simulink model "simulacion"  (R2015a)
settings: Solver=ode45  StartTime=0.0  StopTime=3  RelTol=1e-3
settings Model: Creator=Jesus  LastModifiedBy=Jesus

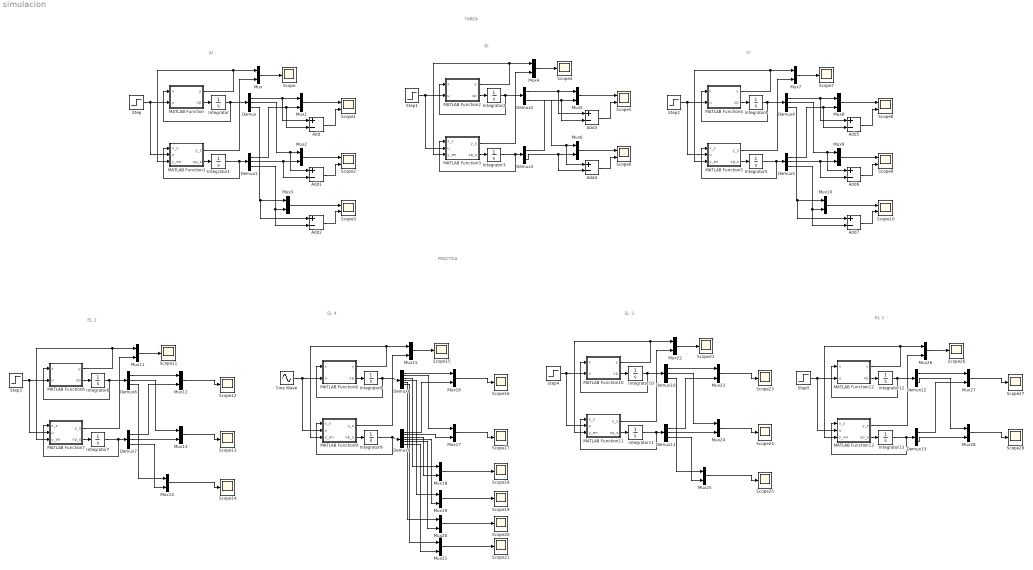
== system simulacion ==
  note: EJ. 4
  note: EJ. 2
  note: PRACTICA
  note: TAREA
  note: A)
  note: B)
  note: C)
  note: EJ. 3
  note: EJ. 1
  Add{,1..7} (8 alike) : Sum  Inputs=+-
  Demux{,1,4..7,10..11} (8 alike) : Demux  Outputs=3
  Demux{2..3,12..13} (4 alike) : Demux  Outputs=2
  Demux8 : Demux  Outputs=6
  Demux9 : Demux  Outputs=6
  Integrator : Integrator  InitialCondition=[3 2 5]
  Integrator{1,5,7,11} (4 alike) : Integrator  InitialCondition=[0 0 0]
  Integrator10 : Integrator  InitialCondition=[3 2 5]
  Integrator12 : Integrator  InitialCondition=[3 5]
  Integrator13 : Integrator  InitialCondition=[0 0]
  Integrator2 : Integrator  InitialCondition=[4 5]
  Integrator3 : Integrator  InitialCondition=[0 0]
  Integrator4 : Integrator  InitialCondition=[10 6 20]
  Integrator6 : Integrator  InitialCondition=[3 2 5]
  Integrator8 : Integrator  InitialCondition=[3 2 5 1 2 3]
  Integrator9 : Integrator  InitialCondition=[0 0 0 0 0 0]
  MATLAB Function : MATLAB Function  TreatAsAtomicUnit=on
  MATLAB Function1 : MATLAB Function  TreatAsAtomicUnit=on
  MATLAB Function10 : MATLAB Function  TreatAsAtomicUnit=on
  MATLAB Function11 : MATLAB Function  TreatAsAtomicUnit=on
  MATLAB Function12 : MATLAB Function  TreatAsAtomicUnit=on
  MATLAB Function13 : MATLAB Function  TreatAsAtomicUnit=on
  MATLAB Function2 : MATLAB Function  TreatAsAtomicUnit=on
  MATLAB Function3 : MATLAB Function  TreatAsAtomicUnit=on
  MATLAB Function4 : MATLAB Function  TreatAsAtomicUnit=on
  MATLAB Function5 : MATLAB Function  TreatAsAtomicUnit=on
  MATLAB Function6 : MATLAB Function  TreatAsAtomicUnit=on
  MATLAB Function7 : MATLAB Function  TreatAsAtomicUnit=on
  MATLAB Function8 : MATLAB Function  TreatAsAtomicUnit=on
  MATLAB Function9 : MATLAB Function  TreatAsAtomicUnit=on
  Mux{,1..28} (29 alike) : Mux  Inputs=2
  Scope{,4,7,11..28} (21 alike) : Scope
      Scope11 settings: SaveName=ScopeData11
      Scope12 settings: SaveName=ScopeData12
      Scope13 settings: SaveName=ScopeData13
      Scope14 settings: SaveName=ScopeData14
      Scope15 settings: SaveName=ScopeData15
      Scope16 settings: SaveName=ScopeData16
      Scope17 settings: YMin=-500000  YMax=5e+06  SaveName=ScopeData17
      Scope18 settings: YMin=-5000  YMax=5000  SaveName=ScopeData18
      Scope19 settings: YMin=-5000  YMax=5000  SaveName=ScopeData19
      Scope20 settings: YMin=-5000  YMax=5000  SaveName=ScopeData20
      Scope21 settings: YMin=-5000  YMax=5000  SaveName=ScopeData21
      Scope22 settings: SaveName=ScopeData22
      Scope23 settings: SaveName=ScopeData23
      Scope24 settings: SaveName=ScopeData24
      Scope25 settings: SaveName=ScopeData25
      Scope26 settings: SaveName=ScopeData26
      Scope27 settings: SaveName=ScopeData27
      Scope28 settings: SaveName=ScopeData28
      Scope4 settings: SaveName=ScopeData4
      Scope7 settings: SaveName=ScopeData8
  Scope{1..3,5..6,8..10} (8 alike) : Scope  NumInputPorts=2
      Scope1 settings: YMin=-5~-5  YMax=5~5
      Scope10 settings: YMin=-5~-5  YMax=5~5  SaveName=ScopeData7
      Scope2 settings: YMin=-5~-5  YMax=5~5  SaveName=ScopeData2
      Scope3 settings: YMin=-5~-5  YMax=5~5  SaveName=ScopeData3
      Scope5 settings: YMin=-5~-5  YMax=5~5  SaveName=ScopeData5
      Scope6 settings: YMin=-5~-5  YMax=5~5  SaveName=ScopeData6
      Scope8 settings: YMin=-5~-5  YMax=5~5  SaveName=ScopeData9
      Scope9 settings: YMin=-5~-5  YMax=5~5  SaveName=ScopeData10
  Sine Wave : Sin  Amplitude=5  SampleTime=0
  Step : Step  SampleTime=0
  Step1 : Step  SampleTime=0
  Step2 : Step  SampleTime=0
  Step3 : Step  After=10  SampleTime=0
  Step4 : Step  After=10  SampleTime=0
  Step5 : Step  After=10  SampleTime=0
  wires:
  MATLAB Function/2(xp) -> Integrator/1
  Integrator/1 -> Demux/1, MATLAB Function/1(x)
  Mux/1 -> Scope/1
  MATLAB Function/1(y) -> MATLAB Function1/3(y_en), Mux/1
  Step/1 -> MATLAB Function1/2(u), MATLAB Function/2(u)
  MATLAB Function1/2(xp_s) -> Integrator1/1
  Integrator1/1 -> MATLAB Function1/1(x_s), Demux1/1
  MATLAB Function1/1(y_s) -> Mux/2
  Demux/1 -> Add/1, Mux1/1
  Demux1/1 -> Add/2, Mux1/2
  Mux1/1 -> Scope1/1
  Mux2/1 -> Scope2/1
  Mux3/1 -> Scope3/1
  Demux/2 -> Add1/1, Mux2/1
  Demux1/2 -> Add1/2, Mux2/2
  Demux/3 -> Add2/1, Mux3/1
  Demux1/3 -> Add2/2, Mux3/2
  Add/1 -> Scope1/2
  Add2/1 -> Scope3/2
  Add1/1 -> Scope2/2
  MATLAB Function2/2(xp) -> Integrator2/1
  Integrator2/1 -> MATLAB Function2/1(x), Demux2/1
  Mux4/1 -> Scope4/1
  MATLAB Function2/1(y) -> Mux4/1, MATLAB Function3/3(y_en)
  Step1/1 -> MATLAB Function2/2(u), MATLAB Function3/2(u)
  MATLAB Function3/2(xp_s) -> Integrator3/1
  Integrator3/1 -> Demux3/1, MATLAB Function3/1(x_s)
  MATLAB Function3/1(y_s) -> Mux4/2
  Demux2/1 -> Mux5/1, Add3/1
  Demux3/1 -> Mux5/2, Add3/2
  Mux5/1 -> Scope5/1
  Mux6/1 -> Scope6/1
  Demux2/2 -> Mux6/1, Add4/1
  Demux3/2 -> Mux6/2, Add4/2
  Add3/1 -> Scope5/2
  Add4/1 -> Scope6/2
  MATLAB Function4/2(xp) -> Integrator4/1
  Integrator4/1 -> MATLAB Function4/1(x), Demux4/1
  Mux7/1 -> Scope7/1
  MATLAB Function4/1(y) -> Mux7/1, MATLAB Function5/3(y_en)
  Step2/1 -> MATLAB Function4/2(u), MATLAB Function5/2(u)
  MATLAB Function5/2(xp_s) -> Integrator5/1
  Integrator5/1 -> Demux5/1, MATLAB Function5/1(x_s)
  MATLAB Function5/1(y_s) -> Mux7/2
  Demux4/1 -> Mux8/1, Add5/1
  Demux5/1 -> Mux8/2, Add5/2
  Mux8/1 -> Scope8/1
  Mux9/1 -> Scope9/1
  Mux10/1 -> Scope10/1
  Demux4/2 -> Mux9/1, Add6/1
  Demux5/2 -> Mux9/2, Add6/2
  Demux4/3 -> Mux10/1, Add7/1
  Demux5/3 -> Mux10/2, Add7/2
  Add5/1 -> Scope8/2
  Add7/1 -> Scope10/2
  Add6/1 -> Scope9/2
  MATLAB Function6/2(xp) -> Integrator6/1
  Integrator6/1 -> MATLAB Function6/1(x), Demux6/1
  Mux11/1 -> Scope11/1
  MATLAB Function6/1(y) -> Mux11/1, MATLAB Function7/3(y_en)
  Step3/1 -> MATLAB Function6/2(u), MATLAB Function7/2(u)
  MATLAB Function7/2(xp_s) -> Integrator7/1
  Integrator7/1 -> Demux7/1, MATLAB Function7/1(x_s)
  MATLAB Function7/1(y_s) -> Mux11/2
  Demux6/1 -> Mux12/1
  Demux7/1 -> Mux12/2
  Mux12/1 -> Scope12/1
  Mux13/1 -> Scope13/1
  Mux14/1 -> Scope14/1
  Demux6/2 -> Mux13/1
  Demux7/2 -> Mux13/2
  Demux6/3 -> Mux14/1
  Demux7/3 -> Mux14/2
  MATLAB Function8/2(xp) -> Integrator8/1
  Integrator8/1 -> Demux8/1, MATLAB Function8/1(x)
  Mux15/1 -> Scope15/1
  MATLAB Function8/1(y) -> MATLAB Function9/3(y_en), Mux15/1
  Sine Wave/1 -> MATLAB Function9/2(u), MATLAB Function8/2(u)
  MATLAB Function9/2(xp_s) -> Integrator9/1
  Integrator9/1 -> MATLAB Function9/1(x_s), Demux9/1
  MATLAB Function9/1(y_s) -> Mux15/2
  Demux8/1 -> Mux16/1
  Demux9/1 -> Mux16/2
  Mux16/1 -> Scope16/1
  Mux17/1 -> Scope17/1
  Mux18/1 -> Scope18/1
  Demux8/2 -> Mux17/1
  Demux9/2 -> Mux17/2
  Demux8/3 -> Mux18/1
  Mux19/1 -> Scope19/1
  Demux8/4 -> Mux19/1
  Demux9/3 -> Mux18/2
  Demux9/4 -> Mux19/2
  Mux20/1 -> Scope20/1
  Demux8/5 -> Mux20/1
  Demux9/5 -> Mux20/2
  Mux21/1 -> Scope21/1
  Demux8/6 -> Mux21/1
  Demux9/6 -> Mux21/2
  MATLAB Function10/2(xp) -> Integrator10/1
  Integrator10/1 -> Demux10/1, MATLAB Function10/1(x)
  Mux22/1 -> Scope22/1
  MATLAB Function10/1(y) -> MATLAB Function11/3(y_en), Mux22/1
  Step4/1 -> MATLAB Function11/2(u), MATLAB Function10/2(u)
  MATLAB Function11/2(xp_s) -> Integrator11/1
  Integrator11/1 -> MATLAB Function11/1(x_s), Demux11/1
  MATLAB Function11/1(y_s) -> Mux22/2
  Demux10/1 -> Mux23/1
  Demux11/1 -> Mux23/2
  Mux23/1 -> Scope23/1
  Mux24/1 -> Scope24/1
  Mux25/1 -> Scope25/1
  Demux10/2 -> Mux24/1
  Demux11/2 -> Mux24/2
  Demux10/3 -> Mux25/1
  Demux11/3 -> Mux25/2
  MATLAB Function12/2(xp) -> Integrator12/1
  Integrator12/1 -> MATLAB Function12/1(x), Demux12/1
  Mux26/1 -> Scope26/1
  MATLAB Function12/1(y) -> Mux26/1, MATLAB Function13/3(y_en)
  Step5/1 -> MATLAB Function12/2(u), MATLAB Function13/2(u)
  MATLAB Function13/2(xp_s) -> Integrator13/1
  Integrator13/1 -> Demux13/1, MATLAB Function13/1(x_s)
  MATLAB Function13/1(y_s) -> Mux26/2
  Demux12/1 -> Mux27/1
  Demux13/1 -> Mux27/2
  Mux27/1 -> Scope27/1
  Mux28/1 -> Scope28/1
  Demux12/2 -> Mux28/1
  Demux13/2 -> Mux28/2

== matlab function simulacion/MATLAB Function1 ==
  data: x_s input; u input; y_s output; xp_s output; y_en input
function [y_s,xp_s] = fcn(x_s,u,y_en)
%#codegen
L=[4 29 10]';
A=[-1 1 -2;0 -1 1;0 0 -1];
B=[1 0 1]';
C=[1 0 0];
xp_s = A*x_s + B*u + L*(y_en-C*x_s);
y_s = C*x_s;

== matlab function simulacion/MATLAB Function ==
  data: x input; u input; y output; xp output
function [y,xp] = fcn(x,u)
%#codegen
A=[-1 1 -2;0 -1 1;0 0 -1];
B=[1 0 1]';
C=[1 0 0];
xp=A*x+B*u;
y = C*x;

== matlab function simulacion/MATLAB Function2 ==
  data: x input; u input; y output; xp output
function [y,xp] = fcn(x,u)
%#codegen
A=[-1 1;1 2];
B=[1 1]';
C=[1 0];
xp=A*x+B*u;
y = C*x;

== matlab function simulacion/MATLAB Function3 ==
  data: x_s input; u input; y_s output; xp_s output; y_en input
function [y_s,xp_s] = fcn(x_s,u,y_en)
%#codegen
L=[11 50]';
A=[-1 1;1 2];
B=[1 1]';
C=[1 0];
xp_s = A*x_s + B*u + L*(y_en-C*x_s);
y_s = C*x_s;

== matlab function simulacion/MATLAB Function4 ==
  data: x input; u input; y output; xp output
function [y,xp] = fcn(x,u)
%#codegen
A=[0 1 0;0 0 1;-5 -6 0];
B=[0 0 1]';
C=[1 0 0];
xp=A*x+B*u;
y = C*x;

== matlab function simulacion/MATLAB Function5 ==
  data: x_s input; u input; y_s output; xp_s output; y_en input
function [y_s,xp_s] = fcn(x_s,u,y_en)
%#codegen
L=[35 394 1285]';
A=[0 1 0;0 0 1;-5 -6 0];
B=[0 0 1]';
C=[1 0 0];
xp_s = A*x_s + B*u + L*(y_en-C*x_s);
y_s = C*x_s;

== matlab function simulacion/MATLAB Function6 ==
  data: x input; u input; y output; xp output
function [y,xp] = fcn(x,u)
%#codegen
A=[0 4 0;-3 0 2;0 0 -2];
B=[0 0 2]';
C=[1 0 0];
xp=A*x+B*u;
y = C*x;

== matlab function simulacion/MATLAB Function7 ==
  data: x_s input; u input; y_s output; xp_s output; y_en input
function [y_s,xp_s] = fcn(x_s,u,y_en)
%#codegen
L=[30 70 87]';
A=[0 4 0;-3 0 2;0 0 -2];
B=[0 0 2]';
C=[1 0 0];
xp_s = A*x_s + B*u + L*(y_en-C*x_s);
y_s = C*x_s;

== matlab function simulacion/MATLAB Function8 ==
  data: x input; u input; y output; xp output
function [y,xp] = fcn(x,u)
%#codegen
A=[0 1 0 0 0 0;16 0 -8 0 0 0;0 0 0 1 0 0;-16 0 16 0 0 0;0 0 0 0 0 1;0 0 0 0 0 0];
B=[0 -1 0 0 0 1]';
C=[1 0 1 0 1 0];
xp=A*x+B*u;
y = C*x;

== matlab function simulacion/MATLAB Function9 ==
  data: x_s input; u input; y_s output; xp_s output; y_en input
function [y_s,xp_s] = fcn(x_s,u,y_en)
%#codegen
L=[-77.3438;-384.3125;90;501.5;2.3438;.8125];
A=[0 1 0 0 0 0;16 0 -8 0 0 0;0 0 0 1 0 0;-16 0 16 0 0 0;0 0 0 0 0 1;0 0 0 0 0 0];
B=[0 -1 0 0 0 1]';
C=[1 0 1 0 1 0];
xp_s = A*x_s + B*u + L*(y_en-C*x_s);
y_s = C*x_s;

== matlab function simulacion/MATLAB Function10 ==
  data: x input; u input; y output; xp output
function [y,xp] = fcn(x,u)
%#codegen
A=[0 1 0;0 0 1;-6 -11 -6];
B=[0 0 1]';
C=[1 0 0];
xp=A*x+B*u;
y = C*x;

== matlab function simulacion/MATLAB Function11 ==
  data: x_s input; u input; y_s output; xp_s output; y_en input
function [y_s,xp_s] = fcn(x_s,u,y_en)
%#codegen
L=[3 7 -1]';
A=[0 1 0;0 0 1;-6 -11 -6];
B=[0 0 1]';
C=[1 0 0];
xp_s = A*x_s + B*u + L*(y_en-C*x_s);
y_s = C*x_s;

== matlab function simulacion/MATLAB Function12 ==
  data: x input; u input; y output; xp output
function [y,xp] = fcn(x,u)
%#codegen
A=[0 1;2 3];
B=[1 1]';
C=[1 2];
xp=A*x+B*u;
y = C*x;

== matlab function simulacion/MATLAB Function13 ==
  data: x_s input; u input; y_s output; xp_s output; y_en input
function [y_s,xp_s] = fcn(x_s,u,y_en)
%#codegen
L=[2 2]';
A=[0 1;2 3];
B=[1 1]';
C=[1 2];
xp_s = A*x_s + B*u + L*(y_en-C*x_s);
y_s = C*x_s;
